simulink model "SWC_TRSP"  (R2020a)
settings: Solver=FixedStepDiscrete  StartTime=0.0  StopTime=0.15  FixedStep=0.0001  RelTol=1e-3
values from neighbouring files (symbols this model uses):
  CAL_TRSP_18VHSVoltCountTrh_s16 = 0.0    [SWC_TRSP_DataDictionary.sldd]
  CAL_TRSP_18VHSVoltDebTrh_s16 = 0.0    [SWC_TRSP_DataDictionary.sldd]
  CAL_TRSP_18VHSVoltErrRst_b = 0.0    [SWC_TRSP_DataDictionary.sldd]
  CAL_TRSP_18VHSVoltHiLim_u16 = 0.0    [SWC_TRSP_DataDictionary.sldd]
  CAL_TRSP_18VHSVoltLoLim_u16 = 0.0    [SWC_TRSP_DataDictionary.sldd]
  CAL_TRSP_1V8CPLDVoltCountTrh_s16 = 0.0    [SWC_TRSP_DataDictionary.sldd]
  CAL_TRSP_1V8CPLDVoltDebTrh_s16 = 0.0    [SWC_TRSP_DataDictionary.sldd]
  CAL_TRSP_1V8CPLDVoltErrRst_b = 0.0    [SWC_TRSP_DataDictionary.sldd]
  CAL_TRSP_1V8CPLDVoltHiLim_u16 = 0.0    [SWC_TRSP_DataDictionary.sldd]
  CAL_TRSP_1V8CPLDVoltLoLim_u16 = 0.0    [SWC_TRSP_DataDictionary.sldd]
  CAL_TRSP_3V3CPLDVoltCountTrh_s16 = 0.0    [SWC_TRSP_DataDictionary.sldd]
  CAL_TRSP_3V3CPLDVoltDebTrh_s16 = 0.0    [SWC_TRSP_DataDictionary.sldd]
  CAL_TRSP_3V3CPLDVoltErrRst_b = 0.0    [SWC_TRSP_DataDictionary.sldd]
  CAL_TRSP_3V3CPLDVoltHiLim_u16 = 0.0    [SWC_TRSP_DataDictionary.sldd]
  CAL_TRSP_3V3CPLDVoltLoLim_u16 = 0.0    [SWC_TRSP_DataDictionary.sldd]
  CAL_TRSP_AgTimecompCtl_u8 = 0.0    [SWC_TRSP_DataDictionary.sldd]
  CAL_TRSP_CurrRngCountTrh_s16 = 0.0    [SWC_TRSP_DataDictionary.sldd]
  CAL_TRSP_CurrRngDebTrh_s16 = 0.0    [SWC_TRSP_DataDictionary.sldd]
  CAL_TRSP_CurrRngErrRst_b = 0.0    [SWC_TRSP_DataDictionary.sldd]
  CAL_TRSP_CurrSumCountTrh_s16 = 0.0    [SWC_TRSP_DataDictionary.sldd]
  CAL_TRSP_CurrSumDebTrh_s16 = 0.0    [SWC_TRSP_DataDictionary.sldd]
  CAL_TRSP_CurrSumErrRst_b = 0.0    [SWC_TRSP_DataDictionary.sldd]
  CAL_TRSP_CurrSumLim_f32 = 0.0    [SWC_TRSP_DataDictionary.sldd]
  CAL_TRSP_Diff_UBR_SBCLim_f32 = 0.0    [SWC_TRSP_DataDictionary.sldd]
  CAL_TRSP_flgChangPha_b = 0.0    [SWC_TRSP_DataDictionary.sldd]
  CAL_TRSP_iPhasSensVoltCountTrh_s16 = 0.0    [SWC_TRSP_DataDictionary.sldd]
  CAL_TRSP_iPhasSensVoltDebTrh_s16 = 0.0    [SWC_TRSP_DataDictionary.sldd]
  CAL_TRSP_iPhasSensVoltErrRst_b = 0.0    [SWC_TRSP_DataDictionary.sldd]
  CAL_TRSP_iPhasSensVoltHiLim_u16 = 0.0    [SWC_TRSP_DataDictionary.sldd]
  CAL_TRSP_iPhasSensVoltLoLim_u16 = 0.0    [SWC_TRSP_DataDictionary.sldd]
  CAL_TRSP_iPhaUOffset_f32 = 0.0    [SWC_TRSP_DataDictionary.sldd]
  CAL_TRSP_iPhaVOffset_f32 = 0.0    [SWC_TRSP_DataDictionary.sldd]
  CAL_TRSP_iPhaWOffset_f32 = 0.0    [SWC_TRSP_DataDictionary.sldd]
  CAL_TRSP_iUCnvFac_f32 = 0.0    [SWC_TRSP_DataDictionary.sldd]
  CAL_TRSP_iVCnvFac_f32 = 0.0    [SWC_TRSP_DataDictionary.sldd]
  CAL_TRSP_iWCnvFac_f32 = 0.0    [SWC_TRSP_DataDictionary.sldd]
  CAL_TRSP_OfstErrRst_b = 0.0    [SWC_TRSP_DataDictionary.sldd]
  CAL_TRSP_OfstRngHiLim_f32 = 0.0    [SWC_TRSP_DataDictionary.sldd]
  CAL_TRSP_OfstRngLoLim_f32 = 0.0    [SWC_TRSP_DataDictionary.sldd]
  CAL_TRSP_ReqTrqCountTrh_s16 = 0.0    [SWC_TRSP_DataDictionary.sldd]
  CAL_TRSP_ReqTrqDebTrh_s16 = 0.0    [SWC_TRSP_DataDictionary.sldd]
  CAL_TRSP_ReqTrqErrRst_b = 0.0    [SWC_TRSP_DataDictionary.sldd]
  CAL_TRSP_ReqTrqHiLim_f32 = 0.0    [SWC_TRSP_DataDictionary.sldd]
  CAL_TRSP_ReqTrqLoLim_f32 = 0.0    [SWC_TRSP_DataDictionary.sldd]
  CAL_TRSP_RslvExciCountTrh_s16 = 0.0    [SWC_TRSP_DataDictionary.sldd]
  CAL_TRSP_RslvExciDebTrh_s16 = 0.0    [SWC_TRSP_DataDictionary.sldd]
  CAL_TRSP_RslvExciErrRst_b = 0.0    [SWC_TRSP_DataDictionary.sldd]
  CAL_TRSP_RslvMaxSele_u8 = 0.0    [SWC_TRSP_DataDictionary.sldd]
  CAL_TRSP_RslvMinSele_u8 = 0.0    [SWC_TRSP_DataDictionary.sldd]
  CAL_TRSP_RslvRngCosNHiLim_u16 = 0.0    [SWC_TRSP_DataDictionary.sldd]
  CAL_TRSP_RslvRngCosNLoLim_u16 = 0.0    [SWC_TRSP_DataDictionary.sldd]
  CAL_TRSP_RslvRngCosPHiLim_u16 = 0.0    [SWC_TRSP_DataDictionary.sldd]
  CAL_TRSP_RslvRngCosPLoLim_u16 = 0.0    [SWC_TRSP_DataDictionary.sldd]
  CAL_TRSP_RslvRngCountTrh_s16 = 0.0    [SWC_TRSP_DataDictionary.sldd]
  CAL_TRSP_RslvRngDebTrh_s16 = 0.0    [SWC_TRSP_DataDictionary.sldd]
  CAL_TRSP_RslvRngErrRst_b = 0.0    [SWC_TRSP_DataDictionary.sldd]
  CAL_TRSP_RslvRngExciHiLim_u16 = 0.0    [SWC_TRSP_DataDictionary.sldd]
  CAL_TRSP_RslvRngExciLoLim_u16 = 0.0    [SWC_TRSP_DataDictionary.sldd]
  CAL_TRSP_RslvRngSinNHiLim_u16 = 0.0    [SWC_TRSP_DataDictionary.sldd]
  CAL_TRSP_RslvRngSinNLoLim_u16 = 0.0    [SWC_TRSP_DataDictionary.sldd]
  CAL_TRSP_RslvRngSinPHiLim_u16 = 0.0    [SWC_TRSP_DataDictionary.sldd]
  CAL_TRSP_RslvRngSinPLoLim_u16 = 0.0    [SWC_TRSP_DataDictionary.sldd]
  CAL_TRSP_RslvSensVoltCountTrh_s16 = 0.0    [SWC_TRSP_DataDictionary.sldd]
  CAL_TRSP_RslvSensVoltDebTrh_s16 = 0.0    [SWC_TRSP_DataDictionary.sldd]
  CAL_TRSP_RslvSensVoltErrRst_b = 0.0    [SWC_TRSP_DataDictionary.sldd]
  CAL_TRSP_RslvSensVoltHiLim_u16 = 0.0    [SWC_TRSP_DataDictionary.sldd]
  CAL_TRSP_RslvSensVoltLoLim_u16 = 0.0    [SWC_TRSP_DataDictionary.sldd]
  CAL_TRSP_RslvSqrtCountTrh_s16 = 0.0    [SWC_TRSP_DataDictionary.sldd]
  CAL_TRSP_RslvSqrtDebTrh_s16 = 0.0    [SWC_TRSP_DataDictionary.sldd]
  CAL_TRSP_RslvSqrtErrRst_b = 0.0    [SWC_TRSP_DataDictionary.sldd]
  CAL_TRSP_RslvSqrtHiLim_u16 = 0.0    [SWC_TRSP_DataDictionary.sldd]
  CAL_TRSP_RslvSqrtLoLim_u16 = 0.0    [SWC_TRSP_DataDictionary.sldd]
  CAL_TRSP_SpeedCtlMode_u8 = 0.0    [SWC_TRSP_DataDictionary.sldd]
  CAL_TRSP_TorqueCtlMode_u8 = 0.0    [SWC_TRSP_DataDictionary.sldd]
  CAL_TRSP_UB_SBCCnvFac_f32 = 0.0    [SWC_TRSP_DataDictionary.sldd]
  CAL_TRSP_UBRVoltCountTrh_s16 = 0.0    [SWC_TRSP_DataDictionary.sldd]
  CAL_TRSP_UBRVoltDebTrh_s16 = 0.0    [SWC_TRSP_DataDictionary.sldd]
  CAL_TRSP_UBRVoltErrRst_b = 0.0    [SWC_TRSP_DataDictionary.sldd]
  CAL_TRSP_UBRWIDECnvFac_f32 = 0.0    [SWC_TRSP_DataDictionary.sldd]
  CAL_TRSP_UCurrRngHiLim_f32 = 0.0    [SWC_TRSP_DataDictionary.sldd]
  CAL_TRSP_UCurrRngLoLim_f32 = 0.0    [SWC_TRSP_DataDictionary.sldd]
  CAL_TRSP_VCurrRngHiLim_f32 = 0.0    [SWC_TRSP_DataDictionary.sldd]
  CAL_TRSP_VCurrRngLoLim_f32 = 0.0    [SWC_TRSP_DataDictionary.sldd]
  CAL_TRSP_WCurrRngHiLim_f32 = 0.0    [SWC_TRSP_DataDictionary.sldd]
  CAL_TRSP_WCurrRngLoLim_f32 = 0.0    [SWC_TRSP_DataDictionary.sldd]
  GLB_TRSP_CircAge_f32 = 0.0    [SWC_TRSP_DataDictionary.sldd]
  GLB_TRSP_MotorPole_u8 = 0.0    [SWC_TRSP_DataDictionary.sldd]
  GLB_TRSP_Sixty_f32 = 0.0    [SWC_TRSP_DataDictionary.sldd]
libraries: simulink x22
(part 4 of 13)

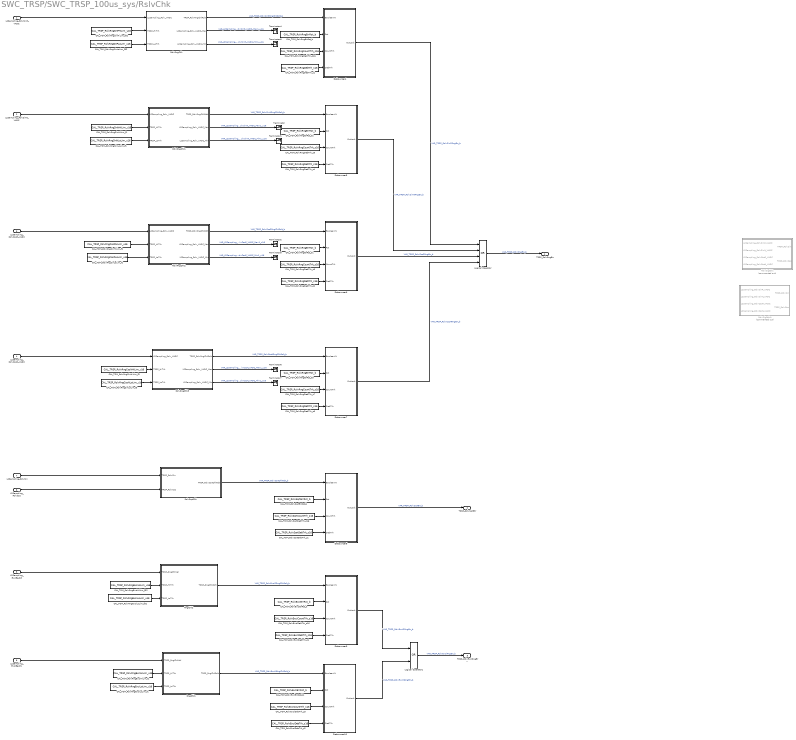
== system SWC_TRSP/SWC_TRSP_100us_sys/RslvChk ==
  L2Sampling_RslvSinP_VADC : Inport
  L2Sampling_RslvSinN_VADC : Inport  Port=2
  L2Sampling_RslvCosP_VADC : Inport  Port=3
  L2Sampling_RslvCosN_VADC : Inport  Port=4
  L2Sampling_ExciBackP : Inport  Port=5
  L2Sampling_ExciBackN : Inport  Port=6
  L2Sampling_RslvSin : Inport  Port=7
  L2Sampling_RslvCos : Inport  Port=8
  CAL_TOM_RslvExciDebTrh_s1 : Constant  Value=CAL_TRSP_RslvExciDebTrh_s16  OutDataTypeStr=int16
  CAL_TOM_RslvExciDebTrh_s16 : Constant  Value=CAL_TRSP_RslvExciCountTrh_s16  OutDataTypeStr=int16
  CAL_TOM_RslvExciDebTrh_s2 : Constant  Value=CAL_TRSP_RslvExciDebTrh_s16  OutDataTypeStr=int16
  CAL_TOM_RslvExciDebTrh_s3 : Constant  Value=CAL_TRSP_RslvExciCountTrh_s16  OutDataTypeStr=int16
  CAL_TOM_RslvExciErrRst_b : Constant  Value=CAL_TRSP_RslvExciErrRst_b  OutDataTypeStr=boolean
  CAL_TOM_RslvExciErrRst_b1 : Constant  Value=CAL_TRSP_RslvExciErrRst_b  OutDataTypeStr=boolean
  CAL_TOM_RslvRngDebTrh_s{1..2,4,6} (4 alike) : Constant  Value=CAL_TRSP_RslvRngDebTrh_s16  OutDataTypeStr=int16
  CAL_TOM_RslvRngDebTrh_s{3,5,7,16} (4 alike) : Constant  Value=CAL_TRSP_RslvRngCountTrh_s16  OutDataTypeStr=int16
  CAL_TOM_RslvRngErrRst_b{,1..3} (4 alike) : Constant  Value=CAL_TRSP_RslvRngErrRst_b  OutDataTypeStr=boolean
  CAL_TOM_RslvRngExciHiLim_f1 : Constant  Value=CAL_TRSP_RslvRngExciHiLim_u16
  CAL_TOM_RslvRngExciHiLim_f32 : Constant  Value=CAL_TRSP_RslvRngExciHiLim_u16
  CAL_TOM_RslvRngExciLoLim_f1 : Constant  Value=CAL_TRSP_RslvRngExciLoLim_u16
  CAL_TOM_RslvRngExciLoLim_f32 : Constant  Value=CAL_TRSP_RslvRngExciLoLim_u16
  CAL_TOM_RslvRngSinHiLim_f1 : Constant  Value=CAL_TRSP_RslvRngSinNHiLim_u16
  CAL_TOM_RslvRngSinHiLim_f2 : Constant  Value=CAL_TRSP_RslvRngCosPHiLim_u16
  CAL_TOM_RslvRngSinHiLim_f3 : Constant  Value=CAL_TRSP_RslvRngCosNHiLim_u16
  CAL_TOM_RslvRngSinHiLim_f32 : Constant  Value=CAL_TRSP_RslvRngSinPHiLim_u16
  CAL_TOM_RslvRngSinLoLim_f1 : Constant  Value=CAL_TRSP_RslvRngSinNLoLim_u16
  CAL_TOM_RslvRngSinLoLim_f2 : Constant  Value=CAL_TRSP_RslvRngCosPLoLim_u16
  CAL_TOM_RslvRngSinLoLim_f3 : Constant  Value=CAL_TRSP_RslvRngCosNLoLim_u16
  CAL_TOM_RslvRngSinLoLim_f32 : Constant  Value=CAL_TRSP_RslvRngSinPLoLim_u16
  CAL_TOM_RslvSqrtDebTrh_s1 : Constant  Value=CAL_TRSP_RslvSqrtDebTrh_s16  OutDataTypeStr=int16
  CAL_TOM_RslvSqrtDebTrh_s16 : Constant  Value=CAL_TRSP_RslvSqrtCountTrh_s16  OutDataTypeStr=int16
  CAL_TOM_RslvSqrtErrRst_b : Constant  Value=CAL_TRSP_RslvSqrtErrRst_b  OutDataTypeStr=boolean
  Debouncer10 : Subsystem  TreatAsAtomicUnit=on
  Debouncer4 : Subsystem  TreatAsAtomicUnit=on
  Debouncer5 : Subsystem  TreatAsAtomicUnit=on
  Debouncer6 : Subsystem  TreatAsAtomicUnit=on
  Debouncer7 : Subsystem  TreatAsAtomicUnit=on
  Debouncer8 : Subsystem  TreatAsAtomicUnit=on
  Debouncer9 : Subsystem  TreatAsAtomicUnit=on
  Logical Operator : Logic  Operator=OR  Inputs=4  AllPortsSameDT=off  OutDataTypeStr=boolean
  Logical Operator1 : Logic  Operator=OR  AllPortsSameDT=off  OutDataTypeStr=boolean
  RngChk1 : Subsystem  TreatAsAtomicUnit=on
  RngChk2 : Subsystem  TreatAsAtomicUnit=on
  RslvRngChk : Subsystem  TreatAsAtomicUnit=on  RTWFcnName=SWC_TRSP_RslvRngChkChk
  RslvRngChk1 : Subsystem  TreatAsAtomicUnit=on  RTWFcnName=SWC_TRSP_RslvRngChkChk
  RslvRngChk2 : Subsystem  TreatAsAtomicUnit=on  RTWFcnName=SWC_TRSP_RslvRngChkChk
  RslvRngChk3 : Subsystem  TreatAsAtomicUnit=on  RTWFcnName=SWC_TRSP_RslvRngChkChk
  RslvSigCalc : Subsystem  Commented=on  TreatAsAtomicUnit=on
      settings: RTWSystemCode=Nonreusable function
  RslvSigCalc1 : Subsystem  Commented=on  TreatAsAtomicUnit=on
      settings: RTWSystemCode=Nonreusable function
  RslvSqrtChk : Subsystem  TreatAsAtomicUnit=on
      settings: RTWSystemCode=Nonreusable function
  Terminator{,1..7} (8 alike) : Terminator
  TRSP_RslvRngErr : Outport
  TRSP_RslvSqrtErr : Outport  Port=2
  TRSP_RslvExciRngErr : Outport  Port=3
  wires:
  CAL_TOM_RslvExciDebTrh_s16/1 -> Debouncer9/3(CountTrh)
  CAL_TOM_RslvExciDebTrh_s1/1 -> Debouncer9/4(DebTrh)
  RngChk2/1(TRSP_RngChkRslt) -> Debouncer9/1(BooleanIN)  "VAR_TRSP_RslvExciPRngChkRslt_b"
  CAL_TOM_RslvExciErrRst_b/1 -> Debouncer9/2(Rst)
  CAL_TOM_RslvSqrtDebTrh_s1/1 -> Debouncer8/4(DebTrh)
  RslvSqrtChk/1(TRSP_RslvSqrtChkRslt) -> Debouncer8/1(BooleanIN)  "VAR_TRSP_RslvSqrtChkRslt_b"
  CAL_TOM_RslvSqrtDebTrh_s16/1 -> Debouncer8/3(CountTrh)
  CAL_TOM_RslvSqrtErrRst_b/1 -> Debouncer8/2(Rst)
  CAL_TOM_RslvRngErrRst_b/1 -> Debouncer4/2(Rst)
  CAL_TOM_RslvRngDebTrh_s1/1 -> Debouncer4/4(DebTrh)
  CAL_TOM_RslvRngDebTrh_s16/1 -> Debouncer4/3(CountTrh)
  RslvRngChk/1(TRSP_RslvRngChkRslt) -> Debouncer4/1(BooleanIN)  "VAR_TRSP_RslvSinPRngChkRslt_b"
  L2Sampling_ExciBackN/1 -> RngChk1/1(TRSP_RngChkVal)
  Debouncer8/1(OutLock) -> TRSP_RslvSqrtErr/1  "VAR_TRSP_RslvSqrtErr_b"
  Debouncer4/1(OutLock) -> Logical Operator/1  "VAR_TRSP_RslvSinPRngErr_b"
  L2Sampling_RslvCosP_VADC/1 -> RslvRngChk2/1(L2Sampling_Rslv_VADC)
  L2Sampling_RslvSinP_VADC/1 -> RslvRngChk/1(L2Sampling_Rslv_VADC)
  Logical Operator1/1 -> TRSP_RslvExciRngErr/1  "VAR_TRSP_RslvExciRngErr_b"
  L2Sampling_ExciBackP/1 -> RngChk2/1(TRSP_RngChkVal)
  Debouncer6/1(OutLock) -> Logical Operator/3  "VAR_TRSP_RslvCosPRngErr_b"
  RslvRngChk2/1(TRSP_RslvRngChkRslt) -> Debouncer6/1(BooleanIN)  "VAR_TRSP_RslvCosPRngChkRslt_b"
  CAL_TOM_RslvRngDebTrh_s3/1 -> Debouncer6/3(CountTrh)
  CAL_TOM_RslvRngDebTrh_s2/1 -> Debouncer6/4(DebTrh)
  CAL_TOM_RslvRngErrRst_b1/1 -> Debouncer6/2(Rst)
  Logical Operator/1 -> TRSP_RslvRngErr/1  "VAR_TRSP_RslvRngErr_b"
  L2Sampling_RslvSinN_VADC/1 -> RslvRngChk1/1(L2Sampling_Rslv_VADC)
  RslvRngChk1/1(TRSP_RslvRngChkRslt) -> Debouncer5/1(BooleanIN)  "VAR_TRSP_RslvSinNRngChkRslt_b"
  CAL_TOM_RslvRngDebTrh_s5/1 -> Debouncer5/3(CountTrh)
  CAL_TOM_RslvRngDebTrh_s4/1 -> Debouncer5/4(DebTrh)
  CAL_TOM_RslvRngErrRst_b2/1 -> Debouncer5/2(Rst)
  CAL_TOM_RslvRngErrRst_b3/1 -> Debouncer7/2(Rst)
  CAL_TOM_RslvRngDebTrh_s6/1 -> Debouncer7/4(DebTrh)
  CAL_TOM_RslvRngDebTrh_s7/1 -> Debouncer7/3(CountTrh)
  RslvRngChk3/1(TRSP_RslvRngChkRslt) -> Debouncer7/1(BooleanIN)  "VAR_TRSP_RslvCosNRngChkRslt_b"
  Debouncer7/1(OutLock) -> Logical Operator/4  "VAR_TRSP_RslvCosNRngErr_b"
  Debouncer5/1(OutLock) -> Logical Operator/2  "VAR_TRSP_RslvSinNRngErr_b"
  CAL_TOM_RslvExciErrRst_b1/1 -> Debouncer10/2(Rst)
  CAL_TOM_RslvExciDebTrh_s2/1 -> Debouncer10/4(DebTrh)
  CAL_TOM_RslvExciDebTrh_s3/1 -> Debouncer10/3(CountTrh)
  RngChk1/1(TRSP_RngChkRslt) -> Debouncer10/1(BooleanIN)  "VAR_TRSP_RslvExciNRngChkRslt_b"
  Debouncer9/1(OutLock) -> Logical Operator1/1  "VAR_TRSP_RslvExciPRngErr_b"
  Debouncer10/1(OutLock) -> Logical Operator1/2  "VAR_TRSP_RslvExciNRngErr_b"
  CAL_TOM_RslvRngExciHiLim_f32/1 -> RngChk2/2(TRSP_HiTrh)
  CAL_TOM_RslvRngExciLoLim_f32/1 -> RngChk2/3(TRSP_LoTrh)
  CAL_TOM_RslvRngExciLoLim_f1/1 -> RngChk1/3(TRSP_LoTrh)
  CAL_TOM_RslvRngExciHiLim_f1/1 -> RngChk1/2(TRSP_HiTrh)
  CAL_TOM_RslvRngSinHiLim_f32/1 -> RslvRngChk/2(TRSP_HiTrh)
  CAL_TOM_RslvRngSinLoLim_f32/1 -> RslvRngChk/3(TRSP_LoTrh)
  CAL_TOM_RslvRngSinHiLim_f1/1 -> RslvRngChk1/2(TRSP_HiTrh)
  CAL_TOM_RslvRngSinLoLim_f1/1 -> RslvRngChk1/3(TRSP_LoTrh)
  CAL_TOM_RslvRngSinLoLim_f2/1 -> RslvRngChk2/3(TRSP_LoTrh)
  CAL_TOM_RslvRngSinHiLim_f2/1 -> RslvRngChk2/2(TRSP_HiTrh)
  CAL_TOM_RslvRngSinHiLim_f3/1 -> RslvRngChk3/2(TRSP_HiTrh)
  CAL_TOM_RslvRngSinLoLim_f3/1 -> RslvRngChk3/3(TRSP_LoTrh)
  L2Sampling_RslvCosN_VADC/1 -> RslvRngChk3/1(L2Sampling_Rslv_VADC)
  RslvRngChk1/2(L2Sampling_Rslv_VADC_Max) -> Terminator/1  "VAR_L2Sampling_RslvSinN_VADC_Max1_u16"
  RslvRngChk1/3(L2Sampling_Rslv_VADC_Min) -> Terminator1/1  "VAR_L2Sampling_RslvSinN_VADC_Min1_u16"
  RslvRngChk2/3(L2Sampling_Rslv_VADC_Min) -> Terminator3/1  "VAR_L2Sampling_RslvCosP_VADC_Min1_u16"
  RslvRngChk2/2(L2Sampling_Rslv_VADC_Max) -> Terminator2/1  "VAR_L2Sampling_RslvCosP_VADC_Max1_u16"
  RslvRngChk/3(L2Sampling_Rslv_VADC_Min) -> Terminator5/1  "VAR_L2Sampling_RslvSinP_VADC_Min1_u16"
  RslvRngChk/2(L2Sampling_Rslv_VADC_Max) -> Terminator4/1  "VAR_L2Sampling_RslvSinP_VADC_Max1_u16"
  RslvRngChk3/2(L2Sampling_Rslv_VADC_Max) -> Terminator6/1  "VAR_L2Sampling_RslvCosN_VADC_Max1_u16"
  RslvRngChk3/3(L2Sampling_Rslv_VADC_Min) -> Terminator7/1  "VAR_L2Sampling_RslvCosN_VADC_Min1_u16"
  L2Sampling_RslvSin/1 -> RslvSqrtChk/1(TRSP_RslvSin)
  L2Sampling_RslvCos/1 -> RslvSqrtChk/2(TRSP_RslvCos)

== system SWC_TRSP/SWC_TRSP_100us_sys/RslvSensVoltChk ==
  L2Sampling_Exci18VLS_MON : Inport
  CAL_TOM_CurrRngDebTrh_s1 : Constant  Value=CAL_TRSP_RslvSensVoltDebTrh_s16  OutDataTypeStr=int16
  CAL_TOM_CurrRngDebTrh_s16 : Constant  Value=CAL_TRSP_RslvSensVoltCountTrh_s16  OutDataTypeStr=int16
  CAL_TOM_CurrRngErrRst_b1 : Constant  Value=CAL_TRSP_RslvSensVoltErrRst_b  OutDataTypeStr=boolean
  CAL_TOM_CurrRngHiLim_f32 : Constant  Value=CAL_TRSP_RslvSensVoltHiLim_u16
  CAL_TOM_CurrRngLoLim_f32 : Constant  Value=CAL_TRSP_RslvSensVoltLoLim_u16
  Debouncer11 : Subsystem  TreatAsAtomicUnit=on
  RngChk : Subsystem  TreatAsAtomicUnit=on
  TRSP_RslvSensVoltRngErr : Outport
  wires:
  CAL_TOM_CurrRngErrRst_b1/1 -> Debouncer11/2(Rst)
  CAL_TOM_CurrRngDebTrh_s16/1 -> Debouncer11/3(CountTrh)
  CAL_TOM_CurrRngDebTrh_s1/1 -> Debouncer11/4(DebTrh)
  RngChk/1(TRSP_RngChkRslt) -> Debouncer11/1(BooleanIN)  "VAR_TRSP_RslvSensVoltRngChkRslt_b"
  L2Sampling_Exci18VLS_MON/1 -> RngChk/1(TRSP_RngChkVal)
  Debouncer11/1(OutLock) -> TRSP_RslvSensVoltRngErr/1  "VAR_TRSP_RslvSensVoltRngErr_b"
  CAL_TOM_CurrRngLoLim_f32/1 -> RngChk/3(TRSP_LoTrh)
  CAL_TOM_CurrRngHiLim_f32/1 -> RngChk/2(TRSP_HiTrh)
